simulink model "stateflow_all"  (R2016b)
settings: Solver=VariableStepAuto  StartTime=0.0  StopTime=10.0  RelTol=1e-3  EnableMultiTasking=on
(part 2 of 2)

== stateflow chart stateflow_all/Chart ==
  state Correct1
    entry:
    a = 0;
    b = 0;
    during:
    a = a + in1;
    b = a * 2;
    state ?
      state State3
        en:
        en_value = 1;
        en_value2 = 2;
        /* 注释不要断行 */
        // 断行用这种符号
      note: en,du,ex都另起一行；
          | 每一行执行语句后一定加分号，不然把结果打印到命令行影响仿真速度;
      note: en语句顶格
      note: 执行语句前面加个空格
      note: 条件语句前不要有空格
      note: 统一在二元运算符前后都加空格
          | 一元运算符不要加，比如b++
      note: 执行语句换行后，加空格
      state State4
        en:
        en_value = 1;
        en_value2 = 2;
        /* 这样断行写,注释就不清楚
        如果中间加入
        en_value2 = a;
        的解释语句的话 */
      note: 各种语句要布置美观，不要超出模块边界
      (default) -> State3
      State3 -> State4 : [a > 0]
          | {
          |  c = b;
          | }
      State4 -> State3 : [a < 1]
    state ?
      note: 4.1 强烈建议 写Action语句时，三个以内的运算符可以写在一行，超出三个则分行写，并注意运算符对齐。
          | 如果涉及到不同运算符，则需要用括号显式注明优先级。
      note: 3.3 强烈建议 状态名与变量名不得相同。
      state Correct
        entry:
        a = 0;
        b = 0;
        during:
        a = a + in1;
        b = a * 2;
      state S10
        during:
        a = a + S10;
        b = a * 2;
        en:
        a = 0;
        ex:
        a = 0;
      note: 4.5 推荐 写执行语句的时候，
          | 前后括号单独在一行，
          | 每一句执行语句各占一行并后加;号。
      note: 3.4 状态内en、du以及ex必须按照这个顺序来写。
          | 如果有组合的比如en,du，则写在最上面或者最下面。
      note: 4.4 严格 注意迁移条件的顺序。
      note: 3.6 建议不要使用exit，如果可以替换成对应的entry。
          | 明确显示出将会在什么状态下执行该语句。
      state B
      Correct -> S10 : % 多个条件写在一行
          | [ condition1 && condition2 && condition3]
      (junction 193) -> Correct [order 1] : {
          |  b = 0;
          | }
      S10 -> (junction 193)
      (junction 193) -> Correct1.?.B [order 2] : [cond2]
    note: 6.3~4 建议同一个 state 最好不要有多个内部跳转。
        | 如果有多个内部跳转，
        | 强烈建议 跳转线按照从上到下的优先级设置。
    Correct1 -> Correct1.? [order 1] : [C1]
    Correct1 -> Correct1.? [order 2] : [C2]
  note: 1.1 强烈建议 所有的 Stateflow 模块的输入输出端口名与对应的信号名相同。
  note: 1.2 强烈建议 未使用的数据不应该留在 Stateflow 模块里。
  note: 1.4 强烈建议 定义Stateflow 变量必须符合以下规范：
      | 所有的局部变量都必须定义在 Chart level及以下； 点我
      | 不同的 chart 之间没有公共变量，除非常数和参数；
      | 嵌套层之间的变量定义不要使用相同名字；
  note: 2.10 数据定义在所使用的状态范围内，除非两个或多个并行状态需要用到同一个数据。
  note: 2.1 强烈建议 跳转箭头不要与其他模型元素交叉、重叠。
  note: 2.6 建议限制单个视图里的状态层数。比如，限制在 3 层以内。
      | 如果超出这个范围，就把内层做成 Subchart ，比如： 点我
      | 2.7 建议限制单个视图内可见的状态个数，一般 6 到 9 个。 点我
      | 2.8 当状态机难以在一个视图上表达清楚时，使用 Subshart 。
      | 2.9 强烈建议 不要为了进行状态分组而滥用并行状态。
  note: 9 事件
      | 9.1 注意 所有的 Event 都必须定义在 chart 层级以及以下，禁止定义在模型层。 不同的chart之间没有local事件的交互。09b以后作为编译错误出现。
      | 9.3 建议 如果触发 Event 的 State 退出时，需要将事件调用的子系统重置， 则建议使用 bind。
      | matlab:ex_bind_fcn_call_subsys_to_state,ex_bind_fcn_call_subsys_to_state
  note: 2.5 必须 取消勾选 'Execute(enter) Chart At Initialization'。
  note: 2.4 强烈建议 默认跳转箭头符合以下规范
      | 位置放在最左上角的明显位置
  state K
    note: 2.2 在任何一层，如果是互斥关系 必须 至少有两个互斥状态以上。
    state KK
      note: 处于状态内部的默认箭头如果连在 Junction 上的话
          | 必须要有一个无条件路径到达某一个状态；
      state B
        en:
        c = b/a;
        note: 2.3 如果使用除法， 建议 要有一定的流程避免除零的情况发生。
      note: 同一层禁止出现多个默认跳转箭头；
      state B2
        en:
      (default) -> (junction 251) [order 2]
      (junction 251) -> K.KK.B [order 1] : [C1]
      (junction 251) -> (junction 253) [order 2]
      K.KK.B -> B2 : send(Event2,KK);
      B2 -> K.KK.B : Event1
      (default) -> B2 [order 1]
      (junction 253) -> B2 : [C2]
    (default) -> KK
    KK -> KK : Event2
  state ?
    note: 3.13 用于状态跳转判断的变量，建议不要使用 du 来更新。
        | 因为 du 语句是在当前跳转判断失败，返回状态后才会执行。
        | 所以会造成，跳转条件满足后延迟一个采样时间步才跳转。
    state Compare1 [parallel]
      settings: executionOrder=1
      state A
      state B
      (default) -> ?.Compare1.A : {
          |  a = 0;
          | }
      ?.Compare1.B -> ?.Compare1.A : {
          |  a = 0;
          | }
      ?.Compare1.A -> (junction 215) : {
          |  a = addOne(a);
          | }
      (junction 215) -> ?.Compare1.B : [ a >= 8]
    state Compare2 [parallel]
      settings: executionOrder=2
      state A
        du:
        b = addOne(b);
      state B
      (default) -> ?.Compare2.A : {
          |  b = 0;
          | }
      ?.Compare2.B -> ?.Compare2.A : {
          |  b = 0;
          | }
      ?.Compare2.A -> ?.Compare2.B : [ b >=8]
  note: 2.11 强烈建议
      | 禁止从外部状态直接跳转到子状态。
  note: 9.2 建议 Event 仅仅为 Function call子系统来使用。
      | 状态转移条件不建议使用 Event。
  note: 5.9 强烈建议禁止对逻辑量进行比较运算
      | 布尔类型的数据禁止与数字(0,1)或者逻辑值(true, false)比较运算。
      | 而是使用 NOT之类的布尔运算符，~ 或者 ！
  note: 5.1 建议 跳转箭头最好要么垂直，要么水平
  note: 5.6 强烈建议 数据比较只在相同数据类型之间进行。
      | 需要对比不同数据类型是，使用显示的数据转换 int16(i)。
  note: 条件语句必须返回布尔量，不要使用非布尔量作为条件
  note: 不允许当 int16_a>float1_a，而indataUint8 == false，
      | 就会产生Backtracking
  note: 5.8 强烈建议
      | 位运算符&，|，^，~
      | 只能用于位运算
  note: 5.2 必须保证没有backtracking.
  note: 5.15 建议不要直接使用函数表达式作为比较值
  note: 9.4 强烈建议 所有时间的广播遵守以下基本原则：
      | 只允许进行方向性的广播事件，使用 send 或者 state.eventname。
      | 如果要广播到多个状态，使用多个 send 语句。
  state y = addOne(x) [function]
    (default) -> (junction 233) : {
        |  y = x + 1;
        | }
  note: 5.7 强烈建议不要直接对比两个浮点数相等。
      | 而是使用差值小于某一个极小值的方式。
      | 直接比较只可用于整形之间。
  note: 10.1 建议 函数函数类型的选用基于以下基本原则：
  state ? [function]
    note: if/then/else 的逻辑
  note: 5.11~13 a++，自加或者自减 必须要单独写为一个 action;
      | 而且在索引里建议不要使用表达式
  note: 5.3~5 建议 不要使用
      | transition Action
      | 强烈建议 不要混用
      | transition Action
      | 和conditon action
  state y = temp_test [function]
    note: 7.1 强烈建议 遵守基本规则：
        | 流程图的条件箭头都水平，动作箭头都竖直，除了循环结构。
        | 箭头语句可以是条件、condition action，不要在流程图里使用 /transition action。
    note: 7.2~4 强烈建议 常见的流程图
        | 使用内置的基本模式。
    note: 8.1 建议 在流程图函数中，
        | 给无条件分支路线增加注释，
        | 显式说明不需要任何动作而不是忘了添加
    note: 8.2~4 建议 只在一个地方给返回值赋值。
        | 另外，流程图里最好只有一个终点Juntion，而且终点 Junction 上只有一条跳转线。
        | 这样就比较清楚的表示出流程图的终点在哪里。
    (junction 146) -> (junction 145) : {
        |  y = 0;
        | }
    (junction 145) -> (junction 144) [order 1] : [ condition1]
    (junction 145) -> (junction 147) [order 2]
    (junction 144) -> (junction 139) : { y = 3;}
    (junction 147) -> (junction 143) [order 1] : [conditon2]
    (junction 147) -> (junction 142) [order 2]
    (junction 143) -> (junction 140) : {y = 2;}
    (junction 142) -> (junction 141) [order 1] : [conditon3]
    (junction 142) -> (junction 138) [order 2]
    (junction 141) -> (junction 137) : { y =1;}
    (junction 139) -> (junction 140)
    (junction 140) -> (junction 137)
    (junction 137) -> (junction 138)
  note: 1.6 建议参数以及常数不要在模型里直接使用数字。
      | 使用 '0'给变量赋初值，或者使用 '1' 作为自增或自减运算除外。
  note: 复杂的方程或者
      |  if/then/else
  state S11
    during:
    a = a + in1;
    b = a * 2;
    note: 6.1 强烈建议 所有的状态的内部跳转连线
        | 必须在 State 框线的左侧面。
    note: 6.2 强烈建立 在 State 内部不要混用
        | en、du,ex等语句和流程图。
        | 因为这样执行顺序不直观。
    note: 作为循环计数器的变量，
        | 在同一个状态内，就只做这一个用途，不要复用。
    note: 5.14 建议在同一个State内不要重用变量
    S11 -> (junction 109) [order 1] : {
        |  i = 1;
        | }
    (junction 109) -> (junction 104) [order 1] : [ i<10]
    (junction 104) -> (junction 101)
    (junction 101) -> (junction 109) : {
        |  i++;
        | }
    (junction 109) -> (junction 107) [order 2] : {
        | i = b + a;
        | }
  state ? [function]
  note: 10.2 建议 是否在 Stateflow 里使用 Simulink 函数时 需要考虑满足这些条件：
      | 只使用到本地的 chart 数据 或者还使用从 simulink 来的输入信号；
      | 被 chart 内的多个地方调用到；
      | 不会每个时间步都调用； stateflow_internalfunction
      | 10.3 建议 不要在内嵌的Simulink里再嵌Stateflow
  note: 传递函数，
      | 积分以及查表
  note: 10.3 一定不要 在 chart 里使用ml.cos(wheelAng)这样语法来调用MATLAB函数
  (default) -> K
  ? -> K.KK.B
  S11 -> Correct1 [order 1] : [ con1 & con2]
  Correct1 -> (junction 92) [order 1] : [boolVar == true]
  (junction 92) -> (junction 89) [order 1] : [ int16_a>float1_a ]
  (junction 89) -> (junction 90) : [ indataUint8]
  (junction 92) -> S11 [order 2] : [ float1 == float2]
      | /{
      |  out = 1;
      | }
  (junction 90) -> S11 : [ tem_test() == 1]
      | {
      |  a = out[k++];
      | }
  data: x function_input double; y function_output double; y function_output double
  events: Event1 local FUNCTION_CALL_EVENT; Event2 local FUNCTION_CALL_EVENT
  function ?:
    | function
